simulink model "EVdemo_6"  (R2013b)
settings: Solver=FixedStepDiscrete  SolverMode=SingleTasking  StartTime=0.0  StopTime=650  FixedStep=4e-5  MaxStep=1e-5  RelTol=1e-3
InitFcn:
  | %EV_Param_Update
  | % update the number of strings (discretized)
  | numStrings = round(Opti_numStrings);
  | %disp(['Number of strings: ' num2str(numStrings)])
  | % update the effective capacity based on the number of strings
  | EV_Param.Battery_Det.Rated_Capacity = 28.5*numStrings; %A*hr
  | EV_Param.Battery_Det.DP = 1.5*fliplr([1500 1500 1600 1450 1325 1125 925 675 425 175 ])./8*EV_Param.Battery_Det.Rated_Capacity; % 8 comes from the 8Ahr rated batter data used (normalize and rescale to the rated capacity
  | EV_Param.Battery_Det.CP = fliplr([25 100 200 250 375 550 750 950 1125 1150])./8*EV_Param.Battery_Det.Rated_Capacity;
  | 
  | % update the number of cells in a string (discretized)
  | numSeriesCells = round(Opti_numSeriesCells);
  | %disp(['Number of cells in a string: ' num2str(numSeriesCells)])
  | % update the nominal string volage and charge deficit
  | EV_Param.Battery_Det.Nominal_Voltage = numSeriesCells*cellVolts;
  | BatteryParams(1).Qe_init = 0;%EV_Param.Battery_Det.Rated_Capacity*(1-EV_Param.Battery_Det.Initial_SOC/100); %Ampere*hours
  | 
  | % update the total number of cells, battery pack mass and total vehicle
  | % mass
  | total_cells = numSeriesCells*numStrings;
  | %disp(['Total Number of cells: ' num2str(total_cells)])
  | EV_Param.BatteryMass = BatteryParams(1).cell_mass*total_cells;
  | %disp(['Total Battery Pack Mass: ' num2str(EV_Param.BatteryMass)])
  | EV_Param.Vehicle.Mass = 1300+EV_Param.BatteryMass;
  | 
  | % update the driveline gear ratio
  | EV_Param.Vehicle.Engine_Vehicle_Gear_Ratio = Opti_Vehicle_Gear_Ratio;
  | %disp(['Driveline gear ratio: ' num2str(Opti_Vehicle_Gear_Ratio)])
StartFcn:
  | %tic;
StopFcn:
  | %toc;
  | %disp([Final SOC: ' num2str(SOC_final)])
  | %disp([Final Vehicle Error: ' num2str(normed_SQE_final)])
model workspace (MAT data in the model file):
  MCOS : class17 (value not decoded)
  MCOS : class17 (value not decoded)
values from neighbouring files (symbols this model uses):
  Drive_Cycle_Num = 8    [startDemo.m]
undefined symbols (not defined in the file or in its folder): Acc_Cmd, BatteryParams, Brake_Set, cell_area, ctrlConst, current_phase_a, Dec_Cmd, direct_current, DiscIntNeverNeededParam, electromagnetic_torque, HEV_Param, Ion, Kt_Temps, Lithium, Mech_Power_kW, Opti_numSeriesCells, Opti_numStrings, Opti_Vehicle_Gear_Ratio, paramVelocityI, paramVelocityP, paramVelocityPICurrentSat, pmsm, quadrature_current, RLoadLoss, rotor_velocity, sigbuilder_block, Ts, Veh_Spd_Ref
libraries: fl_lib x306, nesl_utility x100, LeadAcidBattery_lib x60, simulink x23, powerlib x16, sdl_lib x7, elec_lib x4, electricdrivelib x2, checkpacklib x2, CustomDriveline_lib x2, LiBatteryBlocks x1, Capacitors_lib x1
(part 2 of 7)

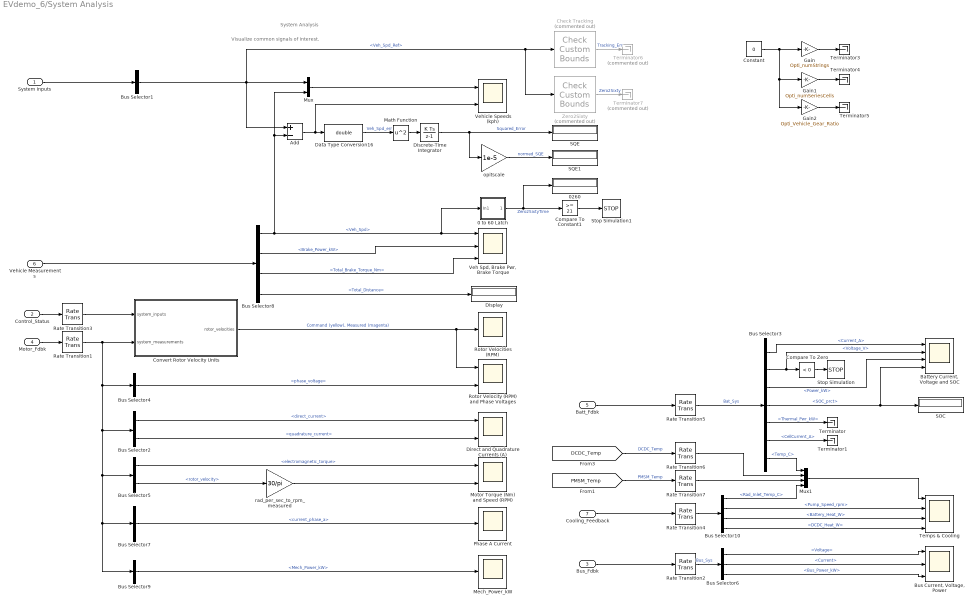
== system EVdemo_6/System Analysis ==
  note: System Analysis
  note: Visualize common signals of interest.
  System Inputs : Inport
  Control_Status : Inport  Port=2
  Bus_Fdbk : Inport  Port=3
  Motor_Fdbk : Inport  Port=4
  Batt_Fdbk : Inport  Port=5
  Vehicle Measurements : Inport  Port=6
  Cooling_Feedback : Inport  Port=7
  0 to 60 Latch : Subsystem
  0260 : Display
  Add : Sum  Inputs=+-
  "Battery Current, Voltage and SOC" : Scope  NumInputPorts=4
      settings: TimeRange=120  YMin=-200~250~-100~93.32  YMax=300~500~100~93.49  SaveName=ScopeData9
  Bus Selector1 : BusSelector  OutputSignals=Veh_Spd_Ref
  Bus Selector10 : BusSelector  OutputSignals=Rad_Inlet_Temp_C,Pump_Speed_rpm,Battery_Heat_W,DCDC_Heat_W
  Bus Selector2 : BusSelector  OutputSignals=Motor_Fdbk.direct_current,Motor_Fdbk.quadrature_current
  Bus Selector3 : BusSelector  OutputSignals=Current_A,Voltage_V,Power_kW,SOC_prct,Thermal_Pwr_kW,CellCurrent_A,Temp_C
  Bus Selector4 : BusSelector  OutputSignals=phase_voltage
  Bus Selector5 : BusSelector  OutputSignals=Motor_Fdbk.electromagnetic_torque,Motor_Fdbk.rotor_velocity
  Bus Selector6 : BusSelector  OutputSignals=Voltage,Current,Bus_Power_kW
  Bus Selector7 : BusSelector  OutputSignals=Motor_Fdbk.current_phase_a
  Bus Selector8 : BusSelector  OutputSignals=Veh_Spd,Brake_Power_kW,Total_Brake_Torque_Nm,Total_Distance
  Bus Selector9 : BusSelector  OutputSignals=Motor_Fdbk.Mech_Power_kW
  "Bus Current, Voltage, Power" : Scope  NumInputPorts=3
      settings: TimeRange=1  YMin=649.5~-40~-14  YMax=655~-12.5~-2  SaveName=ScopeData8
  Check Tracking : checkpacklib/Check Custom Bounds  Commented=on  InstantiateOnLoad=on  enabled=on  stopWhenAssertionFail=off  export=on  ViewDlgPos=[207 433 510 390]  OpenViewOnLoad=off  LaunchViewOnOpen=on  TimeUnits=seconds  EnableUpperBound=off  UpperBoundTimes=[]  UpperBoundAmplitudes=[]  EnableLowerBound=off  LowerBoundTimes=US06_tracking_mat_t  LowerBoundAmplitudes=US06_tracking_mat_lb
  Compare To Constant1 : simulink/Logic and Bit Operations/Compare To Constant  relop=>=  const=21  OutDataTypeStr=boolean
  Compare To Zero : simulink/Logic and Bit Operations/Compare To Zero  relop=<  OutDataTypeStr=boolean
  Constant : Constant  Value=0
  Convert Rotor Velocity Units : Subsystem
  Data Type Conversion16 : DataTypeConversion  OutDataTypeStr=double
  Direct and Quadrature Currents (A) : Scope  NumInputPorts=2
      settings: TimeRange=0.12  YMin=-10~-10  YMax=10~10  SaveName=ScopeData3
  Discrete-Time Integrator : DiscreteIntegrator  SampleTime=-1  ICPrevOutput=DiscIntNeverNeededParam  ICPrevScaledInput=DiscIntNeverNeededParam
  Display : Display
  Gain : Gain  Gain=Opti_numStrings
  Gain1 : Gain  Gain=Opti_numSeriesCells
  Gain2 : Gain  Gain=Opti_Vehicle_Gear_Ratio
  Math Function : Math  Operator=square  SaturateOnIntegerOverflow=on
  Mech_Power_kW : Scope
      settings: TimeRange=2  YMin=-2.5  YMax=27.5  SaveName=ScopeData12
  Motor Torque (Nm) and Speed (RPM) : Scope  NumInputPorts=2
      settings: TimeRange=0.12  YMin=60~-10  YMax=92.5~10  SaveName=ScopeData2
  Mux : Mux  Inputs=2
  Mux1 : Mux
  Phase A Current : Scope
      settings: TimeRange=2  YMin=-400  YMax=400  SaveName=ScopeData11
  Rate Transition{1..7} (7 alike) : RateTransition  OutPortSampleTime=.01
  Rotor Velocities (RPM) : Scope
      settings: TimeRange=2  YMin=3450  YMax=4050
  Rotor Velocity (RPM) and Phase Voltages : Scope  NumInputPorts=2
      settings: TimeRange=1  YMin=-700~-450  YMax=1300~450  SaveName=ScopeData4
  SOC : Display
  SQE : Display
  SQE1 : Display
  Stop Simulation : Stop
  Stop Simulation1 : Stop
  Temps & Cooling : Scope  NumInputPorts=4
      settings: TimeRange=1  YMin=25.75~2289.5~47~-3.75  YMax=29~2295.5~50.25~-1  SaveName=ScopeData5
  Terminator{,1,3..5} (5 alike) : Terminator
  Terminator6 : Terminator  Commented=on
  Terminator7 : Terminator  Commented=on
  "Veh Spd, Brake Pwr, Brake Torque" : Scope  NumInputPorts=3
      settings: TimeRange=1  YMin=617.436~-15~18.25  YMax=682.43~90~18.9  SaveName=ScopeData21
  Vehicle Speeds (kph) : Scope  NumInputPorts=2
      settings: TimeRange=650  YMin=0~-10  YMax=130~130  SaveName=ScopeData6
  Zero2Sixty : checkpacklib/Check Custom Bounds  Commented=on  InstantiateOnLoad=on  enabled=on  stopWhenAssertionFail=off  export=on  ViewDlgPos=[107 568 510 390]  OpenViewOnLoad=off  LaunchViewOnOpen=on  TimeUnits=seconds  EnableUpperBound=off  UpperBoundTimes=[]  UpperBoundAmplitudes=[]  EnableLowerBound=off  LowerBoundTimes=[0 21; 21 22; 22 650]  LowerBoundAmplitudes=[0 0; 97 97; -5 -5]
  opitscale : Gain  Gain=1e-5
  rad_per_sec_to_rpm_measured : Gain  Gain=30/pi
  wires:
  Motor_Fdbk/1 -> Rate Transition1/1
  System Inputs/1 -> Bus Selector1/1
  Convert Rotor Velocity Units/1(rotor_velocities) -> Rotor Velocity (RPM) and Phase Voltages/1, Rotor Velocities (RPM)/1  "Command (yellow), Measured (magenta)"
  Bus Selector2/1 -> Direct and Quadrature Currents (A)/1  "<direct_current>"
  Bus Selector2/2 -> Direct and Quadrature Currents (A)/2  "<quadrature_current>"
  Bus Selector1/1 -> Mux/1, Zero2Sixty/1, Check Tracking/1, Add/1  "<Veh_Spd_Ref>"
  Bus Selector4/1 -> Rotor Velocity (RPM) and Phase Voltages/2  "<phase_voltage>"
  Bus Selector3/4 -> SOC/1, "Battery Current, Voltage and SOC"/4  "<SOC_prct>"
  Bus Selector3/2 -> Compare To Zero/1, "Battery Current, Voltage and SOC"/2  "<Voltage_V>"
  Bus Selector3/1 -> "Battery Current, Voltage and SOC"/1  "<Current_A>"
  Bus Selector5/1 -> Motor Torque (Nm) and Speed (RPM)/1  "<electromagnetic_torque>"
  Bus Selector5/2 -> rad_per_sec_to_rpm_measured/1  "<rotor_velocity>"
  Mux/1 -> Vehicle Speeds (kph)/1
  rad_per_sec_to_rpm_measured/1 -> Motor Torque (Nm) and Speed (RPM)/2
  Bus_Fdbk/1 -> Rate Transition2/1
  Bus Selector6/2 -> "Bus Current, Voltage, Power"/2  "<Current>"
  Bus Selector6/1 -> "Bus Current, Voltage, Power"/1  "<Voltage>"
  Bus Selector7/1 -> Phase A Current/1  "<current_phase_a>"
  Bus Selector8/4 -> Display/1  "<Total_Distance>"
  Bus Selector8/1 -> 0 to 60 Latch/1(In1), "Veh Spd, Brake Pwr, Brake Torque"/1, Mux/2, Add/2  "<Veh_Spd>"
  Bus Selector6/3 -> "Bus Current, Voltage, Power"/3  "<Bus_Power_kW>"
  Bus Selector3/3 -> "Battery Current, Voltage and SOC"/3  "<Power_kW>"
  Bus Selector3/7 -> Mux1/1  "<Temp_C>"
  [DCDC_Temp] -> Rate Transition6/1  "DCDC_Temp"
  Bus Selector9/1 -> Mech_Power_kW/1  "<Mech_Power_kW>"
  Rate Transition5/1 -> Bus Selector3/1  "Bat_Sys"
  Rate Transition2/1 -> Bus Selector6/1  "Bus_Sys"
  Vehicle Measurements/1 -> Bus Selector8/1
  Rate Transition1/1 -> Convert Rotor Velocity Units/2(system_measurements), Bus Selector9/1, Bus Selector7/1, Bus Selector5/1, Bus Selector2/1, Bus Selector4/1
  Control_Status/1 -> Rate Transition3/1
  Batt_Fdbk/1 -> Rate Transition5/1
  Rate Transition3/1 -> Convert Rotor Velocity Units/1(system_inputs)
  Bus Selector3/5 -> Terminator/1  "<Thermal_Pwr_kW>"
  Bus Selector8/2 -> "Veh Spd, Brake Pwr, Brake Torque"/2  "<Brake_Power_kW>"
  Bus Selector8/3 -> "Veh Spd, Brake Pwr, Brake Torque"/3  "<Total_Brake_Torque_Nm>"
  Bus Selector3/6 -> Terminator1/1  "<CellCurrent_A>"
  Add/1 -> Vehicle Speeds (kph)/2, Data Type Conversion16/1
  Discrete-Time Integrator/1 -> SQE/1, opitscale/1  "Squared_Error"
  Data Type Conversion16/1 -> Math Function/1  "Veh_Spd_err"
  opitscale/1 -> SQE1/1  "normed_SQE"
  Cooling_Feedback/1 -> Rate Transition4/1
  Rate Transition4/1 -> Bus Selector10/1
  Bus Selector10/4 -> Temps & Cooling/4  "<DCDC_Heat_W>"
  Bus Selector10/3 -> Temps & Cooling/3  "<Battery_Heat_W>"
  Bus Selector10/2 -> Temps & Cooling/2  "<Pump_Speed_rpm>"
  Bus Selector10/1 -> Mux1/4  "<Rad_Inlet_Temp_C>"
  Rate Transition6/1 -> Mux1/2
  Mux1/1 -> Temps & Cooling/1
  Math Function/1 -> Discrete-Time Integrator/1
  Gain/1 -> Terminator3/1
  Constant/1 -> Gain2/1, Gain1/1, Gain/1
  Gain1/1 -> Terminator4/1
  Gain2/1 -> Terminator5/1
  Compare To Zero/1 -> Stop Simulation/1
  [PMSM_Temp] -> Rate Transition7/1  "PMSM_Temp"
  Rate Transition7/1 -> Mux1/3
  0 to 60 Latch/1(Out1) -> Compare To Constant1/1, 0260/1  "Zero2SixtyTime"
  Compare To Constant1/1 -> Stop Simulation1/1
  Check Tracking/1 -> Terminator6/1  "Tracking_Err"
  Zero2Sixty/1 -> Terminator7/1  "Zero2Sixty"

== system EVdemo_6/Thermal_Partition ==
  Battery Cold Plate : Subsystem
  DCDC Cold Plate : Subsystem
  PMSM Cold Plate : Subsystem
  DCDC_Heat : PMIOPort  Port=1  Side=Left
  Batt_Heat : PMIOPort  Port=2  Side=Left
  PMSM_Heat : PMIOPort  Port=3  Side=Right
  PMSM_Cool : PMIOPort  Port=4  Side=Right
  DCDC_Cool : PMIOPort  Port=5  Side=Right
  Batt_Cool : PMIOPort  Port=6  Side=Right
  connections:
  Battery Cold Plate/LConn1 -- Batt_Heat/RConn1
  DCDC_Heat/RConn1 -- DCDC Cold Plate/LConn1
  PMSM_Heat/RConn1 -- PMSM Cold Plate/LConn1
  DCDC Cold Plate/RConn1 -- DCDC_Cool/RConn1
  Battery Cold Plate/RConn1 -- Batt_Cool/RConn1
  PMSM Cold Plate/RConn1 -- PMSM_Cool/RConn1

== system EVdemo_6/Vehicle ==
  note: 1) Only subsystems can be added as variant choices at this level
      | 2) Blocks cannot be connected at this level as connectivity is
      | automatically determined at simulation, based on the active variant
  System In : Inport
  Grade : Inport  Port=2
  Full : Subsystem  VariantControl=DETAILED_VEHICLE
      mask Display:
      | image('PEV2.jpg');
      | port_label('LConn',1,'Sh');
      | port_label('input',1,'Sys');
  Simple : Subsystem  VariantControl=SYSTEM_VEHICLE  mask(Rigid vehicle model){mass=EV_Param.Vehicle.Mass, area=EV_Param.Vehicle.Frontal_Area, Cd=EV_Param.Vehicle.Aero_Drag_Coeff, radius=EV_Param.Vehicle.Tire_Radius, wheel_inertia=EV_Param.Vehicle.Wheel_Inertia*4, gear_ratio=EV_Param.Vehicle.Engine_Vehicle_Gear_Ratio}
      mask prompts: mass "Vehicle mass (Kg)"; area "Vehicle Area (m^2)"; Cd "Aerodynamic drag coefficient (unitless)"; radius "Tire radius (m)"; wheel_inertia "Total wheel inertia (kg*m^2)"; gear_ratio "Engine to vehicle gear ratio"
      mask help:
      | Model vehicle effective inertia and drag force as seen by the engine. It
      | is assumed that the vehicle is moving on flat terrain. No bearing friction
      | or gear losses are included.
      mask init:
      | gravity = 9.81;
      mask Display:
      | image(imread('HEV_Vehicle_Dynamics_Simple_IMAGE.jpg'));
      | port_label('LConn',1,'Sh');
      | port_label('input',1,'Sys');
  Sh : PMIOPort  Port=1  Side=Left
  Veh_Fdbk : Outport

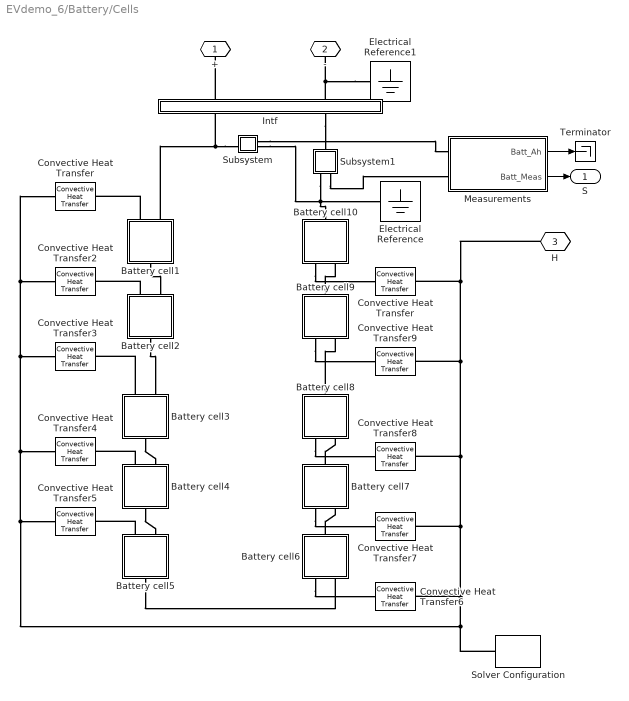
== system EVdemo_6/Battery/Cells ==
  Battery cell1 : Subsystem
      mask Display:
      | image(imread('battery_cell.jpg'))
      | color('red')
      | port_label('LConn',1,'H')
      | port_label('LConn',2,'+')
      | port_label('RConn',1,'-')
  Battery cell10 : Subsystem
      mask Display:
      | image(imread('battery_cell.jpg'))
      | color('red')
      | port_label('LConn',1,'H')
      | port_label('LConn',2,'+')
      | port_label('RConn',1,'-')
  Battery cell2 : Subsystem
      mask Display:
      | image(imread('battery_cell.jpg'))
      | color('red')
      | port_label('LConn',1,'H')
      | port_label('LConn',2,'+')
      | port_label('RConn',1,'-')
  Battery cell3 : Subsystem
      mask Display:
      | image(imread('battery_cell.jpg'))
      | color('red')
      | port_label('LConn',1,'H')
      | port_label('LConn',2,'+')
      | port_label('RConn',1,'-')
  Battery cell4 : Subsystem
      mask Display:
      | image(imread('battery_cell.jpg'))
      | color('red')
      | port_label('LConn',1,'H')
      | port_label('LConn',2,'+')
      | port_label('RConn',1,'-')
  Battery cell5 : Subsystem
      mask Display:
      | image(imread('battery_cell.jpg'))
      | color('red')
      | port_label('LConn',1,'H')
      | port_label('LConn',2,'+')
      | port_label('RConn',1,'-')
  Battery cell6 : Subsystem
      mask Display:
      | image(imread('battery_cell.jpg'))
      | color('red')
      | port_label('LConn',1,'H')
      | port_label('LConn',2,'+')
      | port_label('RConn',1,'-')
  Battery cell7 : Subsystem
      mask Display:
      | image(imread('battery_cell.jpg'))
      | color('red')
      | port_label('LConn',1,'H')
      | port_label('LConn',2,'+')
      | port_label('RConn',1,'-')
  Battery cell8 : Subsystem
      mask Display:
      | image(imread('battery_cell.jpg'))
      | color('red')
      | port_label('LConn',1,'H')
      | port_label('LConn',2,'+')
      | port_label('RConn',1,'-')
  Battery cell9 : Subsystem
      mask Display:
      | image(imread('battery_cell.jpg'))
      | color('red')
      | port_label('LConn',1,'H')
      | port_label('LConn',2,'+')
      | port_label('RConn',1,'-')
  Convective Heat Transfer{,2..9} (9 alike) : fl_lib/Thermal/Thermal Elements/Convective Heat Transfer  area=HEV_Param.Battery_Cell.Area m^2  heat_tr_coeff=HEV_Param.Battery_Cell.Rtheta W/(m^2 * K)  Q_Log=off  T_Log=off  LocalVarNames=|heat_flow|temperature_diff  LocalVarDescs=|Heat flow (J/s)|Temperature difference (K)  LocalVarLogging=[0 0]
  "Convective Heat Transfer " : fl_lib/Thermal/Thermal Elements/Convective Heat Transfer  area=HEV_Param.Battery_Cell.Area m^2  heat_tr_coeff=HEV_Param.Battery_Cell.Rtheta W/(m^2 * K)  Q_Log=off  T_Log=off  LocalVarNames=|heat_flow|temperature_diff  LocalVarDescs=|Heat flow (J/s)|Temperature difference (K)  LocalVarLogging=[0 0]
  Electrical Reference : fl_lib/Electrical/Electrical Elements/Electrical Reference  i_Log=off  LocalVarNames=|i  LocalVarDescs=|i  LocalVarLogging=[]
  Electrical Reference1 : fl_lib/Electrical/Electrical Elements/Electrical Reference  i_Log=off  LocalVarNames=|i  LocalVarDescs=|i  LocalVarLogging=[]
  Intf : Subsystem  mask(Simscape Interface Element){T=100000}
      mask prompts: T "Pole in Transfer Function"
      mask help:
      | Ideal transformer between Simscape circuits.
      |
      | The Voltage across the two terminal pairs are equal and the current flowing through the two branches are equal.
      |
      | The coupling has a transfer function and you need to set the pole in the transfer function.
      mask Display:
      | %color('red');
      | %plot([0.3 0.7],[0.775 0.775]);
      | port_label('LConn', 1,'SPS1')
      | port_label('RConn', 1,'SS1')
      | color('black');
      | %plot([0.3 0.7],[0.225 0.225]);
      | port_label('LConn', 2,'SPS2')
      | port_label('RConn', 2,'SS2')
      | color('green')
      | %text(0.05,0.5,'I Src');
      | color('blue')
      | %text(0.75,0.5,'V Src');
  Measurements : Subsystem
  Solver Configuration : nesl_utility/Solver Configuration  PhysicalDomain=network_engine_domain  SubClassName=solver  LeftPortType=input  RightPortType=generic  Accelerate=off  Tones=[]  Harmonics=[]  SimulateNoise=off  Profile=off  UseLocalSampling=off  EnableSwitchedLinearOptims=on  FrequencyDomain=off  UseCCode=off  RelTol=0.001  AbsTol=1e-06  MinStep=1e-09  ToWorkspace=off  DoDC=off  ResidualTolerance=1e-9  UseLocalSolver=off  LocalSolverChoice=NE_BACKWARD_EULER_ADVANCER  LocalSolverSampleTime=.001  DoFixedCost=off  MaxNonlinIter=3  MaxModeIter=2  LinearAlgebra=Sparse  DelaysMemoryBudget=1024
  Subsystem : Subsystem
      mask Display: disp('S')
  Subsystem1 : Subsystem
      mask Display: disp('S');
  Terminator : Terminator
  + : PMIOPort  Port=1  Side=Right
  - : PMIOPort  Port=2  Side=Right
  H : PMIOPort  Tag=PMCPort  Port=3  Side=Right
  S : Outport
  wires:
  Measurements/2(Batt_Meas) -> S/1
  Measurements/1(Batt_Ah) -> Terminator/1
  connections:
  Electrical Reference1/LConn1 -- -/RConn1 -- Intf/RConn2
  Intf/RConn1 -- +/RConn1
  Intf/LConn2 -- Subsystem1/LConn1
  Subsystem1/RConn2 -- Measurements/LConn2
  Subsystem1/RConn1 -- Battery cell10/RConn1 -- Electrical Reference/LConn1 -- Subsystem/RConn2
  Subsystem/RConn1 -- Measurements/LConn1
  Convective Heat Transfer6/LConn1 -- H/RConn1 -- Convective Heat Transfer/LConn1 -- Convective Heat Transfer9/LConn1 -- Convective Heat Transfer8/LConn1 -- Convective Heat Transfer7/LConn1 -- Solver Configuration/RConn1 -- Convective Heat Transfer2/LConn1 -- "Convective Heat Transfer "/LConn1 -- Convective Heat Transfer3/LConn1 -- Convective Heat Transfer4/LConn1 -- Convective Heat Transfer5/LConn1
  Subsystem/LConn1 -- Intf/LConn1 -- Battery cell1/LConn2
  Battery cell9/LConn1 -- Convective Heat Transfer9/RConn1
  Battery cell8/RConn1 -- Battery cell9/LConn2
  Battery cell8/LConn1 -- Convective Heat Transfer8/RConn1
  Battery cell7/LConn1 -- Convective Heat Transfer7/RConn1
  Battery cell7/RConn1 -- Battery cell8/LConn2
  Battery cell6/LConn1 -- Convective Heat Transfer6/RConn1
  Battery cell6/RConn1 -- Battery cell7/LConn2
  Battery cell5/RConn1 -- Battery cell6/LConn2
  Battery cell5/LConn1 -- Convective Heat Transfer5/RConn1
  Battery cell4/RConn1 -- Battery cell5/LConn2
  Battery cell4/LConn1 -- Convective Heat Transfer4/RConn1
  Battery cell3/RConn1 -- Battery cell4/LConn2
  Battery cell3/LConn1 -- Convective Heat Transfer3/RConn1
  Battery cell2/RConn1 -- Battery cell3/LConn2
  Battery cell9/RConn1 -- Battery cell10/LConn2
  Battery cell2/LConn1 -- Convective Heat Transfer2/RConn1
  Battery cell10/LConn1 -- Convective Heat Transfer/RConn1
  Battery cell1/RConn1 -- Battery cell2/LConn2
  Battery cell1/LConn1 -- "Convective Heat Transfer "/RConn1

== system EVdemo_6/Battery/Electro-Thermal ==
  Controlled Current Source : fl_lib/Electrical/Electrical Sources/Controlled Current Source  i_Log=off  v_Log=off  LocalVarNames=|i|v  LocalVarDescs=|i|v  LocalVarLogging=[0 0]
  Controlled Voltage Source : fl_lib/Electrical/Electrical Sources/Controlled Voltage Source  i_Log=off  v_Log=off  LocalVarNames=|i|v  LocalVarDescs=|i|v  LocalVarLogging=[0 0]
  Current Sensor : fl_lib/Electrical/Electrical Sensors/Current Sensor  i1_Log=off  v1_Log=off  LocalVarNames=|i1|v1  LocalVarDescs=|i1|v1  LocalVarLogging=[0 0]
  Electrical Reference1 : fl_lib/Electrical/Electrical Elements/Electrical Reference  i_Log=off  LocalVarNames=|i  LocalVarDescs=|i  LocalVarLogging=[]
  Lithium Cell : LiBatteryBlocks/Lithium Cell  Battery=BatteryParams(1)
      settings: AttributesFormatString=%<Battery>
  Parallel Strings Divider : fl_lib/Physical Signals/Functions/PS Gain  gain=1/Opti_numStrings  LocalVarLogging=[]
  Series Cells Multiplier : fl_lib/Physical Signals/Functions/PS Gain  gain=Opti_numSeriesCells  LocalVarLogging=[]
  Voltage Sensor : fl_lib/Electrical/Electrical Sensors/Voltage Sensor  i1_Log=off  v1_Log=off  LocalVarNames=|i1|v1  LocalVarDescs=|i1|v1  LocalVarLogging=[0 0]
  + : PMIOPort  Port=1  Side=Right
  - : PMIOPort  Port=2  Side=Right
  H : PMIOPort  Tag=PMCPort  Port=3  Side=Right
  S : Outport
  wires:
  Lithium Cell/1 -> S/1
  connections:
  Voltage Sensor/LConn1 -- Lithium Cell/LConn1 -- Controlled Current Source/LConn1
  Controlled Current Source/RConn2 -- Voltage Sensor/RConn2 -- Lithium Cell/LConn2 -- Electrical Reference1/LConn1
  -/RConn1 -- Controlled Voltage Source/RConn2
  Controlled Voltage Source/RConn1 -- Series Cells Multiplier/RConn1
  Voltage Sensor/RConn1 -- Series Cells Multiplier/LConn1
  Parallel Strings Divider/RConn1 -- Controlled Current Source/RConn1
  Current Sensor/RConn1 -- Parallel Strings Divider/LConn1
  +/RConn1 -- Current Sensor/LConn1
  Current Sensor/RConn2 -- Controlled Voltage Source/LConn1
  Lithium Cell/RConn1 -- H/RConn1

== system EVdemo_6/Battery/Generic ==
  Air Temperature : fl_lib/Physical Signals/Sources/PS Constant  constant=EV_Param.Evniro.Air_Temperature  LocalVarLogging=[]
  Current Sensor : fl_lib/Electrical/Electrical Sensors/Current Sensor  i1_Log=off  v1_Log=off  LocalVarNames=|i1|v1  LocalVarDescs=|i1|v1  LocalVarLogging=[]
  Electrical Reference : fl_lib/Electrical/Electrical Elements/Electrical Reference  i_Log=off  LocalVarNames=|i  LocalVarDescs=|i  LocalVarLogging=[]
  Generic Battery : elec_lib/Sources/Generic Battery  Vnom=HEV_Param.Battery_Sys.Nominal_Voltage V  R1=HEV_Param.Battery_Sys.Internal_Resistance Ohm  prm_AH=2  AH=HEV_Param.Battery_Sys.Rated_Capacity hr*A  AH0=HEV_Param.Battery_Sys.Initial_Charge hr*A  V1=HEV_Param.Battery_Sys.Expn_Voltage V  AH1=HEV_Param.Battery_Sys.Expn_Charge hr*A  prm_R2=1  R2=2e+3 Ohm  LocalVarLogging=[]
  Ideal Temperature Source : fl_lib/Thermal/Thermal Sources/Ideal Temperature Source  Q_Log=off  T_Log=off  LocalVarNames=|Q|T  LocalVarDescs=|Q|T  LocalVarLogging=[0 0]
  Lossy Ultracapacitor : Capacitors_lib/Lossy Ultracapacitor  C0=HEV_Param.UltraCapacitor.Nominal_Capacitance F  Cv=HEV_Param.UltraCapacitor.Rate_C_V F/V  R=HEV_Param.UltraCapacitor.Series_R Ohm  Rd=HEV_Param.UltraCapacitor.Self_Discharge_R Ohm  V0=HEV_Param.UltraCapacitor.Initial_Voltage V  i_Log=off  vc_Log=off  LocalVarNames=|i|v|vc  LocalVarDescs=|Current through variable|Voltage across variable|Internal variable for capacitor voltage  LocalVarLogging=[0 0 0]
  Measurements : Subsystem
  Terminator : Terminator
  Thermal Reference2 : fl_lib/Thermal/Thermal Elements/Thermal Reference  Q_Log=off  LocalVarNames=|Q  LocalVarDescs=|Q  LocalVarLogging=[]
  Voltage Sensor1 : fl_lib/Electrical/Electrical Sensors/Voltage Sensor  i1_Log=off  v1_Log=off  LocalVarNames=|i1|v1  LocalVarDescs=|i1|v1  LocalVarLogging=[]
  + : PMIOPort  Port=1  Side=Right
  - : PMIOPort  Port=2  Side=Right
  H : PMIOPort  Tag=PMCPort  Port=3  Side=Right
  S : Outport
  wires:
  Measurements/2(Batt_Meas) -> S/1
  Measurements/1(Batt_Ah) -> Terminator/1
  connections:
  -/RConn1 -- Current Sensor/LConn1
  Current Sensor/RConn1 -- Measurements/LConn2
  Lossy Ultracapacitor/RConn1 -- Electrical Reference/LConn1 -- Current Sensor/RConn2 -- Voltage Sensor1/RConn2 -- Generic Battery/RConn1
  Lossy Ultracapacitor/LConn1 -- +/RConn1 -- Voltage Sensor1/LConn1 -- Generic Battery/LConn1
  Measurements/LConn1 -- Voltage Sensor1/RConn1
  Ideal Temperature Source/LConn1 -- H/RConn1
  Thermal Reference2/LConn1 -- Ideal Temperature Source/RConn2
  Air Temperature/RConn1 -- Ideal Temperature Source/RConn1

== system EVdemo_6/Battery/Generic1 ==
  Air Temperature : fl_lib/Physical Signals/Sources/PS Constant  constant=EV_Param.Evniro.Air_Temperature  LocalVarLogging=[]
  Current Sensor : fl_lib/Electrical/Electrical Sensors/Current Sensor  i1_Log=off  v1_Log=off  LocalVarNames=|i1|v1  LocalVarDescs=|i1|v1  LocalVarLogging=[]
  Electrical Reference : fl_lib/Electrical/Electrical Elements/Electrical Reference  i_Log=off  LocalVarNames=|i  LocalVarDescs=|i  LocalVarLogging=[]
  Generic Battery : elec_lib/Sources/Generic Battery  Vnom=HEV_Param.Battery_Sys.Nominal_Voltage V  R1=HEV_Param.Battery_Sys.Internal_Resistance Ohm  prm_AH=2  AH=HEV_Param.Battery_Sys.Rated_Capacity hr*A  AH0=HEV_Param.Battery_Sys.Initial_Charge hr*A  V1=HEV_Param.Battery_Sys.Expn_Voltage V  AH1=HEV_Param.Battery_Sys.Expn_Charge hr*A  prm_R2=1  R2=2e+3 Ohm  LocalVarLogging=[]
  Ideal Temperature Source : fl_lib/Thermal/Thermal Sources/Ideal Temperature Source  Q_Log=off  T_Log=off  LocalVarNames=|Q|T  LocalVarDescs=|Q|T  LocalVarLogging=[0 0]
  Measurements : Subsystem
  Terminator : Terminator
  Thermal Reference2 : fl_lib/Thermal/Thermal Elements/Thermal Reference  Q_Log=off  LocalVarNames=|Q  LocalVarDescs=|Q  LocalVarLogging=[]
  Voltage Sensor1 : fl_lib/Electrical/Electrical Sensors/Voltage Sensor  i1_Log=off  v1_Log=off  LocalVarNames=|i1|v1  LocalVarDescs=|i1|v1  LocalVarLogging=[]
  + : PMIOPort  Port=1  Side=Right
  - : PMIOPort  Port=2  Side=Right
  H : PMIOPort  Tag=PMCPort  Port=3  Side=Right
  S : Outport
  wires:
  Measurements/1(Batt_Ah) -> Terminator/1
  Measurements/2(Batt_Meas) -> S/1
  connections:
  Measurements/LConn1 -- Voltage Sensor1/RConn1
  Voltage Sensor1/LConn1 -- Generic Battery/LConn1 -- +/RConn1
  Voltage Sensor1/RConn2 -- Generic Battery/RConn1 -- Electrical Reference/LConn1 -- Current Sensor/RConn2
  Current Sensor/RConn1 -- Measurements/LConn2
  -/RConn1 -- Current Sensor/LConn1
  Thermal Reference2/LConn1 -- Ideal Temperature Source/RConn2
  Air Temperature/RConn1 -- Ideal Temperature Source/RConn1
  Ideal Temperature Source/LConn1 -- H/RConn1

== system EVdemo_6/Battery/Predefined ==
  Air Temperature : fl_lib/Physical Signals/Sources/PS Constant  constant=EV_Param.Evniro.Air_Temperature  LocalVarLogging=[]
  Electrical Reference : fl_lib/Electrical/Electrical Elements/Electrical Reference  Commented=on  i_Log=off  LocalVarNames=|i  LocalVarDescs=|i  LocalVarLogging=0
  GF1 : Subsystem
      mask Display: disp('GF')
  Ground : powerlib/Elements/Ground  Commented=on  LConnTagsString=a
  Ideal Temperature Source : fl_lib/Thermal/Thermal Sources/Ideal Temperature Source  Q_Log=off  T_Log=off  LocalVarNames=|Q|T  LocalVarDescs=|Q|T  LocalVarLogging=[0 0]
  Intf : Subsystem  Commented=on  mask(SimPowerSystems Simscape Interface Element){T=100000}
      mask prompts: T "Pole in Transfer Function"
      mask help:
      | Ideal transformer between a SimPowerSystems circuit and a Simscape circuit.
      |
      | The Voltage across the two terminal pairs are equal and the current flowing through the two branches are equal.
      |
      | The coupling has a transfer function and you need to set the pole in the transfer function.
      mask Display:
      | %color('red');
      | %plot([0.3 0.7],[0.775 0.775]);
      | port_label('LConn', 1,'SPS1')
      | port_label('RConn', 1,'SS1')
      | color('black');
      | %plot([0.3 0.7],[0.225 0.225]);
      | port_label('LConn', 2,'SPS2')
      | port_label('RConn', 2,'SS2')
      | color('green')
      | %text(0.05,0.5,'I Src');
      | color('blue')
      | %text(0.75,0.5,'V Src');
  Preset Battery : electricdrivelib/Extra Sources/Battery  BatType=Lithium-Ion  ShowDetailedParameters=off  NomV=EV_Param.Battery_Det.Nominal_Voltage  NomQ=EV_Param.Battery_Det.Rated_Capacity  SOC=EV_Param.Battery_Det.Initial_SOC  PresetModel=on  MaxQ=85.5  FullV=424.6225  Dis_rate=37.1739  R=0.042667  Normal_OP=77.3217  expZone="[394.1248      4.200652]"  Dis_Char=off  current=[50 100]  Units=Time  Batt_Tr=30
  Thermal Reference2 : fl_lib/Thermal/Thermal Elements/Thermal Reference  Q_Log=off  LocalVarNames=|Q  LocalVarDescs=|Q  LocalVarLogging=[]
  + : PMIOPort  Port=1  Side=Right
  - : PMIOPort  Port=2  Side=Right
  H : PMIOPort  Tag=PMCPort  Port=3  Side=Right
  S : Outport
  wires:
  GF1/1(Out1) -> S/1
  Preset Battery/1 -> GF1/1(In1)
  connections:
  Intf/LConn2 -- Preset Battery/LConn2 -- Ground/LConn1
  Electrical Reference/LConn1 -- -/RConn1 -- Intf/RConn2
  Intf/RConn1 -- +/RConn1
  Intf/LConn1 -- Preset Battery/LConn1
  Thermal Reference2/LConn1 -- Ideal Temperature Source/RConn2
  Air Temperature/RConn1 -- Ideal Temperature Source/RConn1
  Ideal Temperature Source/LConn1 -- H/RConn1

== system EVdemo_6/Battery/RCGeneric ==
  Air Temperature : fl_lib/Physical Signals/Sources/PS Constant  constant=EV_Param.Evniro.Air_Temperature  LocalVarLogging=[]
  C1 : fl_lib/Electrical/Electrical Elements/Capacitor  c=HEV_Param.Battery_Sys.C1.Capacitance F  v0=HEV_Param.Battery_Sys.C1.Initial_Voltage V  r=HEV_Param.Battery_Sys.C1.Series_Resistance Ohm  g=0 1/Ohm  i_Log=off  v_Log=off  vc_Log=off  LocalVarNames=|i|v|vc  LocalVarDescs=|i|v|Internal variable for voltage across capacitor term  LocalVarLogging=[0 0 0]
  Current Sensor : fl_lib/Electrical/Electrical Sensors/Current Sensor  i1_Log=off  v1_Log=off  LocalVarNames=|i1|v1  LocalVarDescs=|i1|v1  LocalVarLogging=[]
  Electrical Reference : fl_lib/Electrical/Electrical Elements/Electrical Reference  i_Log=off  LocalVarNames=|i  LocalVarDescs=|i  LocalVarLogging=[]
  Generic Battery : elec_lib/Sources/Generic Battery  Vnom=HEV_Param.Battery_Sys.Nominal_Voltage V  R1=HEV_Param.Battery_Sys.Internal_Resistance Ohm  prm_AH=2  AH=HEV_Param.Battery_Sys.Rated_Capacity hr*A  AH0=HEV_Param.Battery_Sys.Initial_Charge hr*A  V1=HEV_Param.Battery_Sys.Expn_Voltage V  AH1=HEV_Param.Battery_Sys.Expn_Charge hr*A  prm_R2=1  R2=2e+3 Ohm  LocalVarLogging=[]
  Ideal Temperature Source : fl_lib/Thermal/Thermal Sources/Ideal Temperature Source  Q_Log=off  T_Log=off  LocalVarNames=|Q|T  LocalVarDescs=|Q|T  LocalVarLogging=[0 0]
  Measurements : Subsystem
  R1 : fl_lib/Electrical/Electrical Elements/Resistor  R=HEV_Param.Battery_Sys.R1 Ohm  i_Log=off  v_Log=off  LocalVarNames=|i|v  LocalVarDescs=|i|v  LocalVarLogging=[0 0]
  R2 : fl_lib/Electrical/Electrical Elements/Resistor  R=HEV_Param.Battery_Sys.R2 Ohm  i_Log=off  v_Log=off  LocalVarNames=|i|v  LocalVarDescs=|i|v  LocalVarLogging=[0 0]
  Terminator : Terminator
  Thermal Reference2 : fl_lib/Thermal/Thermal Elements/Thermal Reference  Q_Log=off  LocalVarNames=|Q  LocalVarDescs=|Q  LocalVarLogging=[]
  Voltage Sensor1 : fl_lib/Electrical/Electrical Sensors/Voltage Sensor  i1_Log=off  v1_Log=off  LocalVarNames=|i1|v1  LocalVarDescs=|i1|v1  LocalVarLogging=[]
  + : PMIOPort  Port=1  Side=Right
  - : PMIOPort  Port=2  Side=Right
  H : PMIOPort  Tag=PMCPort  Port=3  Side=Right
  S : Outport
  wires:
  Measurements/2(Batt_Meas) -> S/1
  Measurements/1(Batt_Ah) -> Terminator/1
  connections:
  Generic Battery/LConn1 -- R1/RConn1
  C1/RConn1 -- R1/LConn1 -- R2/RConn1
  -/RConn1 -- Current Sensor/LConn1
  Current Sensor/RConn1 -- Measurements/LConn2
  Current Sensor/RConn2 -- Electrical Reference/LConn1 -- Generic Battery/RConn1 -- Voltage Sensor1/RConn2
  C1/LConn1 -- R2/LConn1 -- Voltage Sensor1/LConn1 -- +/RConn1
  Measurements/LConn1 -- Voltage Sensor1/RConn1
  Thermal Reference2/LConn1 -- Ideal Temperature Source/RConn2
  Air Temperature/RConn1 -- Ideal Temperature Source/RConn1
  Ideal Temperature Source/LConn1 -- H/RConn1

== system EVdemo_6/Bus Sensors/LPF ==
  In : Inport
  Discrete-Time Integrator2 : DiscreteIntegrator  IntegratorMethod=Integration: Trapezoidal  SampleTime=-1  ShowStatePort=on  ICPrevOutput=DiscIntNeverNeededParam  ICPrevScaledInput=DiscIntNeverNeededParam
  FixPt Data Type Duplicate1 : DataTypeDuplicate  DisableCoverage=on  NumInputPorts=3
  Sum : Sum  Inputs=|+-
  w : Gain  Gain=w
  Out : Outport
  wires:
  Discrete-Time Integrator2/State -> Sum/2
  Sum/1 -> w/1
  Discrete-Time Integrator2/1 -> Out/1, FixPt Data Type Duplicate1/1
  In/1 -> Sum/1, FixPt Data Type Duplicate1/3
  w/1 -> Discrete-Time Integrator2/1, FixPt Data Type Duplicate1/2

== system EVdemo_6/Bus Sensors/LPF1 ==
  In : Inport
  Discrete-Time Integrator2 : DiscreteIntegrator  IntegratorMethod=Integration: Trapezoidal  SampleTime=-1  ShowStatePort=on  ICPrevOutput=DiscIntNeverNeededParam  ICPrevScaledInput=DiscIntNeverNeededParam
  FixPt Data Type Duplicate1 : DataTypeDuplicate  DisableCoverage=on  NumInputPorts=3
  Sum : Sum  Inputs=|+-
  w : Gain  Gain=w
  Out : Outport
  wires:
  w/1 -> FixPt Data Type Duplicate1/2, Discrete-Time Integrator2/1
  In/1 -> FixPt Data Type Duplicate1/3, Sum/1
  Discrete-Time Integrator2/1 -> FixPt Data Type Duplicate1/1, Out/1
  Sum/1 -> w/1
  Discrete-Time Integrator2/State -> Sum/2

== system EVdemo_6/Cooling System/Charge_Accumulator ==
  Accumulator : fl_lib/Thermal Liquid/Elements/Translational Mechanical Converter (TL)  or=1  interface_area=pi/4*.01^2 m^2  x0=0.1 m  dead_volume=1e-3 m^3  T0=BatteryParams(1).T_init K  dynamic_compressibility=0  p0=1 atm  LocalVarLogging=[]
  Bar2F : fl_lib/Physical Signals/Functions/PS Gain  gain=pi/4*.01^2*1e5  LocalVarLogging=[]
  Charge Pressure : fl_lib/Physical Signals/Sources/PS Constant  constant=3  LocalVarLogging=[]
  Ideal Force Source : fl_lib/Mechanical/Mechanical Sources/Ideal Force Source  v_Log=off  f_Log=off  LocalVarNames=|v|f  LocalVarDescs=|v|f  LocalVarLogging=[0 0]
  Mechanical Translational Reference : fl_lib/Mechanical/Translational Elements/Mechanical Translational Reference  f_Log=off  LocalVarNames=|f  LocalVarDescs=|f  LocalVarLogging=0
  Mechanical Translational Reference1 : fl_lib/Mechanical/Translational Elements/Mechanical Translational Reference  f_Log=off  LocalVarNames=|f  LocalVarDescs=|f  LocalVarLogging=0
  Perfect Insulator : fl_lib/Thermal/Thermal Elements/Perfect Insulator  LocalVarLogging=[]
  Port : PMIOPort  Port=1  Side=Left
  connections:
  Mechanical Translational Reference1/LConn1 -- Ideal Force Source/LConn1
  Charge Pressure/RConn1 -- Bar2F/LConn1
  Bar2F/RConn1 -- Ideal Force Source/RConn1
  Mechanical Translational Reference/LConn1 -- Accumulator/LConn2
  Accumulator/RConn1 -- Ideal Force Source/RConn2
  Perfect Insulator/LConn1 -- Accumulator/LConn3
  Port/RConn1 -- Accumulator/LConn1

== system EVdemo_6/Cooling System/Cooling Pump And Control ==
  Cooling_Pump : fl_lib/Thermal Liquid/Sources/Controlled Mass Flow Rate Source (TL)  length=5e-2 m  area=.01*.04 m^2  mdot_A_Log=off  mdot_B_Log=off  Phi_A_Log=off  Phi_convection_A_Log=off  Phi_B_Log=off  Phi_convection_B_Log=off  T_Log=off  p_Log=off  u_Log=off  u_A_Log=off  u_B_Log=off  rho_Log=off  rho_A_Log=off  rho_B_Log=off  cp_Log=off  alpha_Log=off  k_Log=off  beta_Log=off  nu_Log=off  LocalVarNames=|mdot_A|mdot_B|Phi_A|Phi_convection_A|Phi_B|Phi_convection_B|T|p|u|u_A|u_B|rho|rho_A|rho_B|cp|alpha|k|beta|nu  LocalVarDescs=|Incoming Mass Flow Rate into port A|Incoming Mass Flow Rate into port B|Incoming Thermal Flux through port A|Convective part of incoming Thermal Flux through port A|Incoming Thermal Flux through port B|Convective part of incoming Thermal Flux through port B|Temperature inside the component|Pressure inside the component|u|u_A|u_B|rho|rho_A|rho_B|cp|alpha|k|beta|nu  LocalVarLogging=[0 0 0 0 0 0 0 0 0 0 0 0 0 0 0 0 0 0 0]
  PS Constant : fl_lib/Physical Signals/Sources/PS Constant  constant=272.15  LocalVarLogging=[]
  PS Subtract : fl_lib/Physical Signals/Functions/PS Subtract  LocalVarLogging=[]
  PS-Simulink Converter : nesl_utility/PS-Simulink Converter  PhysicalDomain=network_engine_domain  SubClassName=ps_output  LeftPortType=input  RightPortType=output  PseudoPeriodic=off  Frequencies=[]  Unit=1  AffineConversion=off
  Relay : Relay  OnSwitchValue=40  OffSwitchValue=30
  Temp2rpm : fl_lib/Physical Signals/Lookup Tables/PS Lookup Table (1D)  x_t=[280 300 320 340]  y_t=[0 2500 3500 3800]  interp_method=1  extrap_method=1  LocalVarLogging=[]
  Unit Delay : UnitDelay  SampleTime=-1
  rpm2radps*roh*D : fl_lib/Physical Signals/Functions/PS Gain  gain=pi/30*1000*5e-6  LocalVarLogging=[]
  Inlet : PMIOPort  Port=1  Side=Left
  Pump_Speed_rpm : PMIOPort  Port=2  Side=Right
  Temp : PMIOPort  Port=3  Side=Right
  Temp_Fedbk : PMIOPort  Port=4  Side=Left
  Outlet : PMIOPort  Port=5  Side=Right
  Fan_Cmd : Outport
  wires:
  PS-Simulink Converter/1 -> Unit Delay/1
  Relay/1 -> Fan_Cmd/1
  Unit Delay/1 -> Relay/1
  connections:
  Cooling_Pump/RConn1 -- Outlet/RConn1
  rpm2radps*roh*D/RConn1 -- Cooling_Pump/LConn2
  Temp2rpm/RConn1 -- Pump_Speed_rpm/RConn1 -- rpm2radps*roh*D/LConn1
  Cooling_Pump/LConn1 -- Inlet/RConn1
  Temp_Fedbk/RConn1 -- PS Subtract/LConn1 -- Temp2rpm/LConn1
  PS Subtract/RConn1 -- PS-Simulink Converter/LConn1 -- Temp/RConn1
  PS Constant/RConn1 -- PS Subtract/LConn2

== system EVdemo_6/Cooling System/Fan ==
  Fan_Cmd : Inport
  Air Temp : fl_lib/Physical Signals/Sources/PS Constant  constant=BatteryParams(1).T_init  LocalVarLogging=[]
  Controlled Convective Heat Transfer : CustomThermal_lib/Controlled Convective Heat Transfer  area=.5*.5 m^2  heat_tr_coeff_min=0 W/(m^2 * K)  Q_Log=off  T_Log=off  LocalVarNames=|Q|T  LocalVarDescs=|Q|T  LocalVarLogging=[0 0]
  Ideal Heat Flow Sensor : fl_lib/Thermal/Thermal Sensors/Ideal Heat Flow Sensor  Q_Log=off  T_Log=off  LocalVarNames=|Q|T  LocalVarDescs=|Q|T  LocalVarLogging=[0 0]
  Ideal Temperature Source : fl_lib/Thermal/Thermal Sources/Ideal Temperature Source  Q_Log=off  T_Log=off  LocalVarNames=|heat_flow|T_differential  LocalVarDescs=|Heat flow rate through the source (J/s)|Temperature differential across the source (K)  LocalVarLogging=[0 0]
  PS-Simulink Converter1 : nesl_utility/PS-Simulink Converter  PhysicalDomain=network_engine_domain  SubClassName=ps_output  LeftPortType=input  RightPortType=output  PseudoPeriodic=off  Frequencies=[]  Unit=W  AffineConversion=on
  Rate Limiter : RateLimiter  RisingSlewLimit=50  FallingSlewLimit=-50  SampleTimeMode=inherited  InitialCondition=15
  Scope : Scope
      settings: YMin=4.07  YMax=4.2  SaveName=ScopeData10
  Simulink-PS Converter : nesl_utility/Simulink-PS Converter  PhysicalDomain=network_engine_domain  SubClassName=ps_input  LeftPortType=input  RightPortType=output  PseudoPeriodic=off  Frequencies=[]  NoiseDistribution=none  NoiseParameters=[]  Unit=1  AffineConversion=off  InputFiltering=off  SimscapeFilterOrder=1  InputFilterTimeConstant=0.001  UdotUserProvided=1
  Switch : Switch  Criteria=u2 > Threshold
  Therm Ref : fl_lib/Thermal/Thermal Elements/Thermal Reference  Q_Log=off  LocalVarNames=|Q  LocalVarDescs=|Q  LocalVarLogging=[]
  h_Fan_Off : Constant  Value=15  SampleTime=-1
  h_Fan_On : Constant  Value=200  SampleTime=-1
  Rad_Port : PMIOPort  Port=1  Side=Right
  wires:
  h_Fan_On/1 -> Switch/1
  h_Fan_Off/1 -> Switch/3
  Switch/1 -> Rate Limiter/1
  Rate Limiter/1 -> Simulink-PS Converter/1
  Fan_Cmd/1 -> Switch/2
  PS-Simulink Converter1/1 -> Scope/1
  connections:
  Simulink-PS Converter/RConn1 -- Controlled Convective Heat Transfer/LConn2  "Rad_Convection"
  Air Temp/RConn1 -- Ideal Temperature Source/RConn1
  Therm Ref/LConn1 -- Ideal Temperature Source/RConn2
  Ideal Heat Flow Sensor/LConn1 -- Controlled Convective Heat Transfer/LConn1
  Controlled Convective Heat Transfer/RConn1 -- Rad_Port/RConn1
  Ideal Heat Flow Sensor/RConn1 -- PS-Simulink Converter1/LConn1
  Ideal Heat Flow Sensor/RConn2 -- Ideal Temperature Source/LConn1

== system EVdemo_6/Cooling System/Temp Probe ==
  Absolute Reference (TL) : fl_lib/Thermal Liquid/Elements/Absolute Reference (TL)  mdot_Log=off  Phi_Log=off  LocalVarNames=|mdot|Phi  LocalVarDescs=|mdot|Phi  LocalVarLogging=[0 0]
  "Pressure & Temperature Sensor " : fl_lib/Thermal Liquid/Sensors/Pressure & Temperature Sensor (TL)  mdot_Log=off  Phi_Log=off  LocalVarNames=|mdot|Phi  LocalVarDescs=|mdot|Phi  LocalVarLogging=[0 0]
  Conn1 : PMIOPort  Port=1  Side=Left
  Conn3 : PMIOPort  Port=2  Side=Right
  connections:
  Absolute Reference (TL)/LConn1 -- "Pressure & Temperature Sensor "/RConn1
  "Pressure & Temperature Sensor "/RConn3 -- Conn1/RConn1
  "Pressure & Temperature Sensor "/LConn1 -- Conn3/RConn1
